simulink model "SOLTEST"  (R2026a)
settings: Solver=ode23t  StopTime=T_sweep*1.01  MaxStep=1e-3
InitFcn:
  | init_params
values from neighbouring files (symbols this model uses):
  G_cell = 1000 * ones(Ns,1)    [init_params.m]
  T_sweep = 1    [init_params.m]
  V_oc = 22.8    [init_params.m]
libraries: nesl_utility x45, pv_lib x37, fl_lib x8, ee_lib x3, simulink x2
settings Model: Creator=cdt  LastModifiedBy=cdt

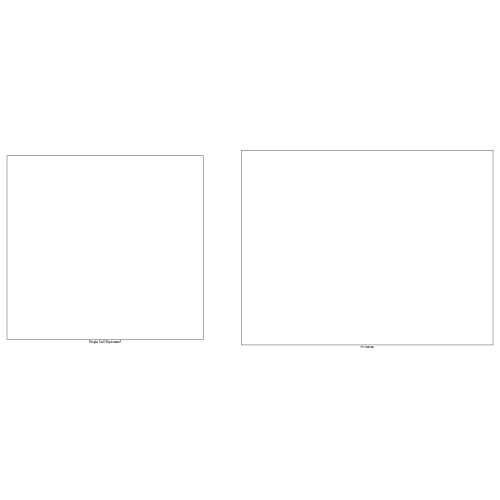
[thumbnail: Simulink's stored preview of the top-level diagram]
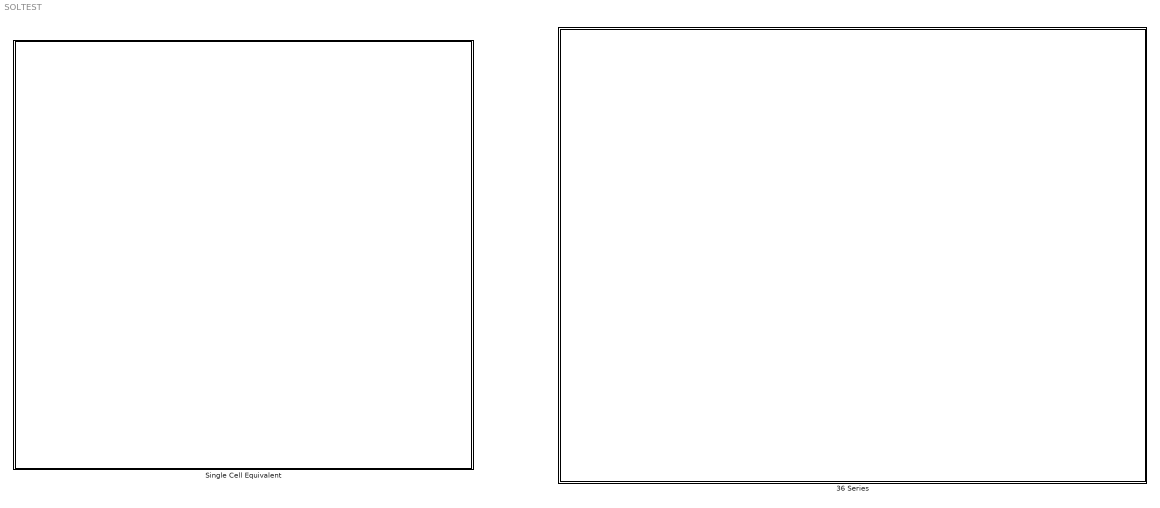
== system SOLTEST ==
  36 Series : Subsystem
  Single Cell Equivalent : Subsystem

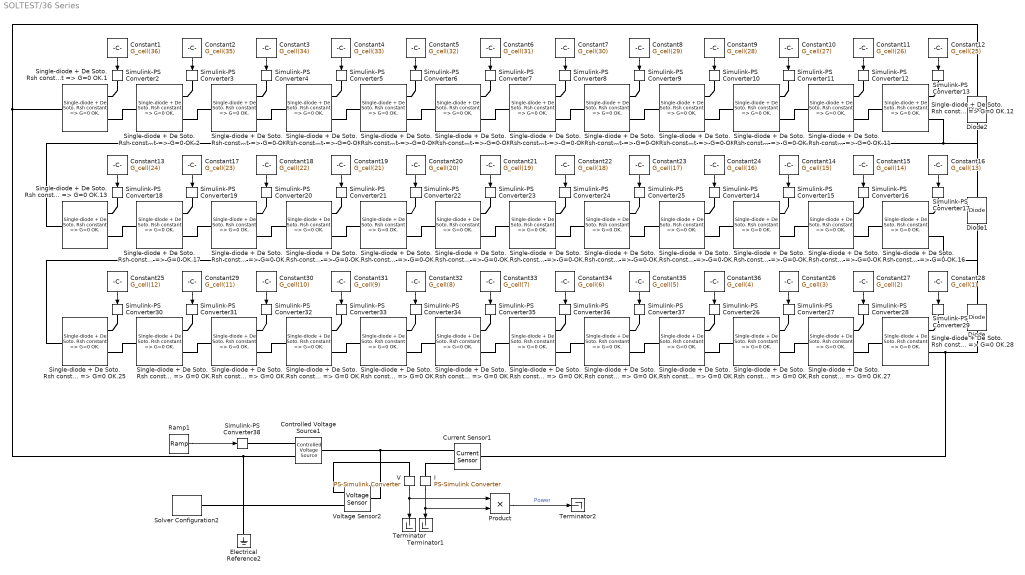
== system SOLTEST/36 Series ==
  Constant1 : Constant  Value=G_cell(36)
  Constant10 : Constant  Value=G_cell(27)
  Constant11 : Constant  Value=G_cell(26)
  Constant12 : Constant  Value=G_cell(25)
  Constant13 : Constant  Value=G_cell(24)
  Constant14 : Constant  Value=G_cell(15)
  Constant15 : Constant  Value=G_cell(14)
  Constant16 : Constant  Value=G_cell(13)
  Constant17 : Constant  Value=G_cell(23)
  Constant18 : Constant  Value=G_cell(22)
  Constant19 : Constant  Value=G_cell(21)
  Constant2 : Constant  Value=G_cell(35)
  Constant20 : Constant  Value=G_cell(20)
  Constant21 : Constant  Value=G_cell(19)
  Constant22 : Constant  Value=G_cell(18)
  Constant23 : Constant  Value=G_cell(17)
  Constant24 : Constant  Value=G_cell(16)
  Constant25 : Constant  Value=G_cell(12)
  Constant26 : Constant  Value=G_cell(3)
  Constant27 : Constant  Value=G_cell(2)
  Constant28 : Constant  Value=G_cell(1)
  Constant29 : Constant  Value=G_cell(11)
  Constant3 : Constant  Value=G_cell(34)
  Constant30 : Constant  Value=G_cell(10)
  Constant31 : Constant  Value=G_cell(9)
  Constant32 : Constant  Value=G_cell(8)
  Constant33 : Constant  Value=G_cell(7)
  Constant34 : Constant  Value=G_cell(6)
  Constant35 : Constant  Value=G_cell(5)
  Constant36 : Constant  Value=G_cell(4)
  Constant4 : Constant  Value=G_cell(33)
  Constant5 : Constant  Value=G_cell(32)
  Constant6 : Constant  Value=G_cell(31)
  Constant7 : Constant  Value=G_cell(30)
  Constant8 : Constant  Value=G_cell(29)
  Constant9 : Constant  Value=G_cell(28)
  Controlled Voltage Source1 : fl_lib/Electrical/Electrical Sources/Controlled Voltage Source
  Current Sensor1 : fl_lib/Electrical/Electrical Sensors/Current Sensor
  Diode : ee_lib/Semiconductors & Converters/Diode  ModelType=ee.enum.diode.modelType.pwl  TableType=ee.enum.diode.tableType.IfMat  IfMat=[.07, .12, .19, 1.75, 4.24, 7.32, 11.2; .16, .3, .72, 2.14, 5.02, 8.35, 13.12] A  VfMat=[.9, 1.15, 1.25, 1.5, 1.75, 2.17, 2.6, 2.85; .58, .68, .75, 1.1, 1.38, 1.77, 2.27, 2.7] V  TjVec=[25, 125] degC  VfVec=[.5, .7, .9, 1.3, 1.7, 2.1, 2.5] V  IfVec=[.1, .2, .5, 1, 2, 4, 7, 10] A  IrMat=[1e-06, 2e-06, 5e-06, 1e-05, 2.5e-05, 5e-05, .0001; 2e-06, 5e-06, 1e-05, 4e-05, 8e-05, .0002, .0005] A  VrMat=[10, 100, 200, 250, 300, 325, 350; 10, 70, 160, 220, 270, 300, 320] V  VrVec=[10, 20, 40, 50, 70, 80, 100] V  IrVec=[1e-06, 2e-06, 5e-06, 1e-05, 2e-05, 5e-05, .0001] A  Vf=0.2 V  Ron=0.3 Ohm  Goff=1e-8 S  prmExp=ee.enum.diode.expParam.useTwo  I12=[.0137, .545] A  V12=[.6, .7] V  RS=0 Ohm  Tmeas=298.15 K  IS=1e-12 A  ec=1  I1=0.0137 A  V1=0.6 V  N_series=1  N_parallel=1  ZenerEnable=false  Rz=0.3 Ohm  BV=30 V  C_param=ee.enum.diode.capParam.fixed  CJ=0 pF  CJ0=5 pF  Vvec=[.1, 10, 100] V  Cvec=[3.5, 1, .4] pF  VJ=1 V  Mgrad=0.5  FC=0.5  Q_param=ee.enum.diode.recoveryParam.off  iRM=-7.15 A  iF=4 A  didt=-750 A/us  trr_factor=3  trr=115 ns  Qrr=150 nA*s  Vr=-600 V  Ls=150 nH  Erec=0.03 J  TT=50 ns  tau=100 ns  T_param=ee.enum.diode.temperatureParam.off  Tdevice=298.15 K  I1_T2=0.245 A  V1_T2=0.5 V  IS_T2=1.25e-7 A  Tmeas2=125 degC  XTI_param=ee.enum.diode.xtiParam.pn  XTI=3  EG_param=ee.enum.diode.egapParam.material_si  EG=1.11 eV  dBVdT=0 V/K  enable_fault_input=simscape.enum.onoff.off  i_specify=off  i_priority=None  i=0 A  i_nominal_specify=off  i_nominal_value=1  i_nominal_unit=A  v_specify=off  v_priority=None  v=0 V  v_nominal_specify=off  v_nominal_value=1  v_nominal_unit=V  v_capacitor_specify=off  v_capacitor_priority=None  v_capacitor=0 V  v_capacitor_nominal_specify=off  v_capacitor_nominal_value=1  v_capacitor_nominal_unit=V  Qj_specify=off  Qj_priority=High  Qj=0 C  Qj_nominal_specify=off  Qj_nominal_value=1  Qj_nominal_unit=C  i_diode_specify=off  i_diode_priority=None  i_diode=0 A  i_diode_nominal_specify=off  i_diode_nominal_value=1  i_diode_nominal_unit=A  v_diode_specify=off  v_diode_priority=None  v_diode=0 V  v_diode_nominal_specify=off  v_diode_nominal_value=1  v_diode_nominal_unit=V  i_capacitor_specify=off  i_capacitor_priority=None  i_capacitor=0 A  i_capacitor_nominal_specify=off  i_capacitor_nominal_value=1  i_capacitor_nominal_unit=A  fidelity_level=ee.enum.diode.fidelity.includeChargeDyn  rec_loss_model=ee.enum.diode.reverseRecoveryModelTabulateUpTo3D.fixed  ErecVal=0 J  scaleWithIandV=true  ErecMat=zeros(2, 3) J  ErecMat3D=zeros(2, 3, 2) J  TjrecVec=[298.15, 398.15] K  IfrecVec=[.1, 1, 10] A  IrecVal=10 A  VrecVal=10 V  VrecVec=[0, 100] V  tFilter=1 / 1000 / 100 s  thermal_network_parameterization=ee.enum.thermalNetworkTopology.junctionCase  Rth=[0, 10] K/W  Rth_Cauer=[1, 3, 10] K/W  Rth_Foster=[.08, .14, .22, .16] K/W  thermal_mass_parameterization=ee.enum.thermalNetwork.timeconstant  thermal_mass=[0, 1] J/K  thermal_mass_Cauer=[.1, .3, 1] J/K  thermal_mass_Foster=[.001, .005, .05, .5] J/K  thermal_time_constant=[0, 10] s  thermal_time_constant_Cauer=[1, 3, 10] s  thermal_time_constant_Foster=[7e-05, .0007, .01, .08] s  thermal_mass_initial_temperatures=[25, 25] degC  thermal_mass_initial_temperatures_Cauer=[25, 25, 25] degC  junction_thermal_mass=0.01 J/K  Tvec_initial_Foster=[25, 25, 25, 25] degC  no_thermal_network=0  junction_temperature_specify=off  junction_temperature_priority=None  junction_temperature=25 degC  junction_temperature_nominal_specify=off  junction_temperature_nominal_value=1  junction_temperature_nominal_unit=degC
  Diode1 : ee_lib/Semiconductors & Converters/Diode  ModelType=ee.enum.diode.modelType.pwl  TableType=ee.enum.diode.tableType.IfMat  IfMat=[.07, .12, .19, 1.75, 4.24, 7.32, 11.2; .16, .3, .72, 2.14, 5.02, 8.35, 13.12] A  VfMat=[.9, 1.15, 1.25, 1.5, 1.75, 2.17, 2.6, 2.85; .58, .68, .75, 1.1, 1.38, 1.77, 2.27, 2.7] V  TjVec=[25, 125] degC  VfVec=[.5, .7, .9, 1.3, 1.7, 2.1, 2.5] V  IfVec=[.1, .2, .5, 1, 2, 4, 7, 10] A  IrMat=[1e-06, 2e-06, 5e-06, 1e-05, 2.5e-05, 5e-05, .0001; 2e-06, 5e-06, 1e-05, 4e-05, 8e-05, .0002, .0005] A  VrMat=[10, 100, 200, 250, 300, 325, 350; 10, 70, 160, 220, 270, 300, 320] V  VrVec=[10, 20, 40, 50, 70, 80, 100] V  IrVec=[1e-06, 2e-06, 5e-06, 1e-05, 2e-05, 5e-05, .0001] A  Vf=0.2 V  Ron=0.3 Ohm  Goff=1e-8 S  prmExp=ee.enum.diode.expParam.useTwo  I12=[.0137, .545] A  V12=[.6, .7] V  RS=0 Ohm  Tmeas=298.15 K  IS=1e-12 A  ec=1  I1=0.0137 A  V1=0.6 V  N_series=1  N_parallel=1  ZenerEnable=false  Rz=0.3 Ohm  BV=30 V  C_param=ee.enum.diode.capParam.fixed  CJ=0 pF  CJ0=5 pF  Vvec=[.1, 10, 100] V  Cvec=[3.5, 1, .4] pF  VJ=1 V  Mgrad=0.5  FC=0.5  Q_param=ee.enum.diode.recoveryParam.off  iRM=-7.15 A  iF=4 A  didt=-750 A/us  trr_factor=3  trr=115 ns  Qrr=150 nA*s  Vr=-600 V  Ls=150 nH  Erec=0.03 J  TT=50 ns  tau=100 ns  T_param=ee.enum.diode.temperatureParam.off  Tdevice=298.15 K  I1_T2=0.245 A  V1_T2=0.5 V  IS_T2=1.25e-7 A  Tmeas2=125 degC  XTI_param=ee.enum.diode.xtiParam.pn  XTI=3  EG_param=ee.enum.diode.egapParam.material_si  EG=1.11 eV  dBVdT=0 V/K  enable_fault_input=simscape.enum.onoff.off  i_specify=off  i_priority=None  i=0 A  i_nominal_specify=off  i_nominal_value=1  i_nominal_unit=A  v_specify=off  v_priority=None  v=0 V  v_nominal_specify=off  v_nominal_value=1  v_nominal_unit=V  v_capacitor_specify=off  v_capacitor_priority=None  v_capacitor=0 V  v_capacitor_nominal_specify=off  v_capacitor_nominal_value=1  v_capacitor_nominal_unit=V  Qj_specify=off  Qj_priority=High  Qj=0 C  Qj_nominal_specify=off  Qj_nominal_value=1  Qj_nominal_unit=C  i_diode_specify=off  i_diode_priority=None  i_diode=0 A  i_diode_nominal_specify=off  i_diode_nominal_value=1  i_diode_nominal_unit=A  v_diode_specify=off  v_diode_priority=None  v_diode=0 V  v_diode_nominal_specify=off  v_diode_nominal_value=1  v_diode_nominal_unit=V  i_capacitor_specify=off  i_capacitor_priority=None  i_capacitor=0 A  i_capacitor_nominal_specify=off  i_capacitor_nominal_value=1  i_capacitor_nominal_unit=A  fidelity_level=ee.enum.diode.fidelity.includeChargeDyn  rec_loss_model=ee.enum.diode.reverseRecoveryModelTabulateUpTo3D.fixed  ErecVal=0 J  scaleWithIandV=true  ErecMat=zeros(2, 3) J  ErecMat3D=zeros(2, 3, 2) J  TjrecVec=[298.15, 398.15] K  IfrecVec=[.1, 1, 10] A  IrecVal=10 A  VrecVal=10 V  VrecVec=[0, 100] V  tFilter=1 / 1000 / 100 s  thermal_network_parameterization=ee.enum.thermalNetworkTopology.junctionCase  Rth=[0, 10] K/W  Rth_Cauer=[1, 3, 10] K/W  Rth_Foster=[.08, .14, .22, .16] K/W  thermal_mass_parameterization=ee.enum.thermalNetwork.timeconstant  thermal_mass=[0, 1] J/K  thermal_mass_Cauer=[.1, .3, 1] J/K  thermal_mass_Foster=[.001, .005, .05, .5] J/K  thermal_time_constant=[0, 10] s  thermal_time_constant_Cauer=[1, 3, 10] s  thermal_time_constant_Foster=[7e-05, .0007, .01, .08] s  thermal_mass_initial_temperatures=[25, 25] degC  thermal_mass_initial_temperatures_Cauer=[25, 25, 25] degC  junction_thermal_mass=0.01 J/K  Tvec_initial_Foster=[25, 25, 25, 25] degC  no_thermal_network=0  junction_temperature_specify=off  junction_temperature_priority=None  junction_temperature=25 degC  junction_temperature_nominal_specify=off  junction_temperature_nominal_value=1  junction_temperature_nominal_unit=degC
  Diode2 : ee_lib/Semiconductors & Converters/Diode  ModelType=ee.enum.diode.modelType.pwl  TableType=ee.enum.diode.tableType.IfMat  IfMat=[.07, .12, .19, 1.75, 4.24, 7.32, 11.2; .16, .3, .72, 2.14, 5.02, 8.35, 13.12] A  VfMat=[.9, 1.15, 1.25, 1.5, 1.75, 2.17, 2.6, 2.85; .58, .68, .75, 1.1, 1.38, 1.77, 2.27, 2.7] V  TjVec=[25, 125] degC  VfVec=[.5, .7, .9, 1.3, 1.7, 2.1, 2.5] V  IfVec=[.1, .2, .5, 1, 2, 4, 7, 10] A  IrMat=[1e-06, 2e-06, 5e-06, 1e-05, 2.5e-05, 5e-05, .0001; 2e-06, 5e-06, 1e-05, 4e-05, 8e-05, .0002, .0005] A  VrMat=[10, 100, 200, 250, 300, 325, 350; 10, 70, 160, 220, 270, 300, 320] V  VrVec=[10, 20, 40, 50, 70, 80, 100] V  IrVec=[1e-06, 2e-06, 5e-06, 1e-05, 2e-05, 5e-05, .0001] A  Vf=0.2 V  Ron=0.3 Ohm  Goff=1e-8 S  prmExp=ee.enum.diode.expParam.useTwo  I12=[.0137, .545] A  V12=[.6, .7] V  RS=0 Ohm  Tmeas=298.15 K  IS=1e-12 A  ec=1  I1=0.0137 A  V1=0.6 V  N_series=1  N_parallel=1  ZenerEnable=false  Rz=0.3 Ohm  BV=30 V  C_param=ee.enum.diode.capParam.fixed  CJ=0 pF  CJ0=5 pF  Vvec=[.1, 10, 100] V  Cvec=[3.5, 1, .4] pF  VJ=1 V  Mgrad=0.5  FC=0.5  Q_param=ee.enum.diode.recoveryParam.off  iRM=-7.15 A  iF=4 A  didt=-750 A/us  trr_factor=3  trr=115 ns  Qrr=150 nA*s  Vr=-600 V  Ls=150 nH  Erec=0.03 J  TT=50 ns  tau=100 ns  T_param=ee.enum.diode.temperatureParam.off  Tdevice=298.15 K  I1_T2=0.245 A  V1_T2=0.5 V  IS_T2=1.25e-7 A  Tmeas2=125 degC  XTI_param=ee.enum.diode.xtiParam.pn  XTI=3  EG_param=ee.enum.diode.egapParam.material_si  EG=1.11 eV  dBVdT=0 V/K  enable_fault_input=simscape.enum.onoff.off  i_specify=off  i_priority=None  i=0 A  i_nominal_specify=off  i_nominal_value=1  i_nominal_unit=A  v_specify=off  v_priority=None  v=0 V  v_nominal_specify=off  v_nominal_value=1  v_nominal_unit=V  v_capacitor_specify=off  v_capacitor_priority=None  v_capacitor=0 V  v_capacitor_nominal_specify=off  v_capacitor_nominal_value=1  v_capacitor_nominal_unit=V  Qj_specify=off  Qj_priority=High  Qj=0 C  Qj_nominal_specify=off  Qj_nominal_value=1  Qj_nominal_unit=C  i_diode_specify=off  i_diode_priority=None  i_diode=0 A  i_diode_nominal_specify=off  i_diode_nominal_value=1  i_diode_nominal_unit=A  v_diode_specify=off  v_diode_priority=None  v_diode=0 V  v_diode_nominal_specify=off  v_diode_nominal_value=1  v_diode_nominal_unit=V  i_capacitor_specify=off  i_capacitor_priority=None  i_capacitor=0 A  i_capacitor_nominal_specify=off  i_capacitor_nominal_value=1  i_capacitor_nominal_unit=A  fidelity_level=ee.enum.diode.fidelity.includeChargeDyn  rec_loss_model=ee.enum.diode.reverseRecoveryModelTabulateUpTo3D.fixed  ErecVal=0 J  scaleWithIandV=true  ErecMat=zeros(2, 3) J  ErecMat3D=zeros(2, 3, 2) J  TjrecVec=[298.15, 398.15] K  IfrecVec=[.1, 1, 10] A  IrecVal=10 A  VrecVal=10 V  VrecVec=[0, 100] V  tFilter=1 / 1000 / 100 s  thermal_network_parameterization=ee.enum.thermalNetworkTopology.junctionCase  Rth=[0, 10] K/W  Rth_Cauer=[1, 3, 10] K/W  Rth_Foster=[.08, .14, .22, .16] K/W  thermal_mass_parameterization=ee.enum.thermalNetwork.timeconstant  thermal_mass=[0, 1] J/K  thermal_mass_Cauer=[.1, .3, 1] J/K  thermal_mass_Foster=[.001, .005, .05, .5] J/K  thermal_time_constant=[0, 10] s  thermal_time_constant_Cauer=[1, 3, 10] s  thermal_time_constant_Foster=[7e-05, .0007, .01, .08] s  thermal_mass_initial_temperatures=[25, 25] degC  thermal_mass_initial_temperatures_Cauer=[25, 25, 25] degC  junction_thermal_mass=0.01 J/K  Tvec_initial_Foster=[25, 25, 25, 25] degC  no_thermal_network=0  junction_temperature_specify=off  junction_temperature_priority=None  junction_temperature=25 degC  junction_temperature_nominal_specify=off  junction_temperature_nominal_value=1  junction_temperature_nominal_unit=degC
  Electrical Reference2 : fl_lib/Electrical/Electrical Elements/Electrical Reference
  I : nesl_utility/PS-Simulink Converter  PhysicalDomain=network_engine_domain  SubClassName=ps_output  LeftPortType=input  RightPortType=output  PseudoPeriodic=off  Frequencies=[]  VectorFormat=inherit  Unit=inherit  AffineConversion=off
  Product : Product
  Ramp1 : simulink/Sources/Ramp  slope=V_oc/T_sweep  start=0  InitialOutput=0
  Simulink-PS Converter{2..37} (36 alike) : nesl_utility/Simulink-PS Converter  PhysicalDomain=network_engine_domain  SubClassName=ps_input  LeftPortType=input  RightPortType=output  PseudoPeriodic=off  Frequencies=[]  NoiseDistribution=none  NoiseParameters=[]  Unit=W/m^2  AffineConversion=off  FilteringAndDerivatives=provide  SimscapeFilterOrder=1  InputFilterTimeConstant=0.001  UdotUserProvided=0
  Simulink-PS Converter38 : nesl_utility/Simulink-PS Converter  PhysicalDomain=network_engine_domain  SubClassName=ps_input  LeftPortType=input  RightPortType=output  PseudoPeriodic=off  Frequencies=[]  NoiseDistribution=none  NoiseParameters=[]  Unit=1  AffineConversion=off  FilteringAndDerivatives=provide  SimscapeFilterOrder=1  InputFilterTimeConstant=0.001  UdotUserProvided=0
  Single-diode + De Soto. Rsh constant => G=0 OK.{1..36} (36 alike) : pv_lib/Single-diode + De Soto. Rsh constant => G=0 OK.  IL_ref=IL_ref A  I0_ref=I0_ref A  a_ref=a_ref V  Rs=Rs Ohm  Rsh_ref=Rsh_ref Ohm  alpha=alpha A/K  T=298.15 K  Gref=1000 W/m^2  Tref=298.15 K  Eg_ref=1.121 eV  dEgdT=0.0002677 1/K  kB=8.617333262e-5 eV/K  i_specify=off  i_priority=None  i=0 A  i_nominal_specify=off  i_nominal_value=1  i_nominal_unit=A  v_specify=off  v_priority=None  v=0 V  v_nominal_specify=off  v_nominal_value=1  v_nominal_unit=V
  Solver Configuration2 : nesl_utility/Solver Configuration  PhysicalDomain=network_engine_domain  SubClassName=solver  LeftPortType=input  RightPortType=generic  Tones=[]  Harmonics=[]  SimulateNoise=off  Profile=off  UseLocalSampling=off  EnableSwitchedLinearOptims=on  FrequencyDomain=off  UseCCode=off  RelTol=0.001  AbsTol=0.001  MinStep=1e-09  ToWorkspace=off  RevertToSquareIcSolve=off  NumHomotopyIterations=100  PhasorMode=off  PhasorModeNumHarmonics=1  ConsistencySolver=NEWTON_XTOL_AFTER_FTOL  CanonicalOrdering=CANONICAL  OptimizeIntermediates=OPTIMIZED  IndexReductionMethod=DerivativeReplacement  DoDC=off  ResidualTolerance=1e-09  ConsistencyTolSource=GLOBAL  ConsistencyAbsTol=0.001  ConsistencyRelTol=0.001  ConsistencyTolFactor=0.001  UseLocalSolver=off  LocalSolverChoice=NE_BACKWARD_EULER_ADVANCER  ResolveIndetEquations=on  FunctionEvalNumThread=1  LocalSolverSampleTime=0.001  DoFixedCost=off  MaxNonlinIter=3  MaxModeIter=2  ComputeImpulses=off  ImpulseIterations=2  LinearAlgebra=auto  LinearAlgebraNumThread=0  EquationFormulation=NE_TIME_EF  DelaysMemoryBudget=1024  AutomaticFiltering=on  FilteringTimeConstant=0.001  PartitionStorageMethod=AS_NEEDED  PartitionMemoryBudget=1024  PartitionMethod=ROBUST  MultibodyUseLocalSolver=off  MultibodyLocalSolverChoice=ODE1  MultibodyLocalSolverSampleTime=0.001
  Terminator : Terminator
  Terminator1 : Terminator
  Terminator2 : Terminator
  V : nesl_utility/PS-Simulink Converter  PhysicalDomain=network_engine_domain  SubClassName=ps_output  LeftPortType=input  RightPortType=output  PseudoPeriodic=off  Frequencies=[]  VectorFormat=inherit  Unit=inherit  AffineConversion=off
  Voltage Sensor2 : fl_lib/Electrical/Electrical Sensors/Voltage Sensor
  wires:
  Constant25/1 -> Simulink-PS Converter30/1
  Constant14/1 -> Simulink-PS Converter15/1
  I/1 -> Product/2, Terminator1/1
  Constant33/1 -> Simulink-PS Converter35/1
  Constant9/1 -> Simulink-PS Converter10/1
  Ramp1/1 -> Simulink-PS Converter38/1
  V/1 -> Product/1, Terminator/1
  Constant19/1 -> Simulink-PS Converter21/1
  Constant29/1 -> Simulink-PS Converter31/1
  Constant11/1 -> Simulink-PS Converter12/1
  Constant3/1 -> Simulink-PS Converter4/1
  Constant35/1 -> Simulink-PS Converter37/1
  Constant31/1 -> Simulink-PS Converter33/1
  Constant36/1 -> Simulink-PS Converter26/1
  Constant22/1 -> Simulink-PS Converter24/1
  Constant5/1 -> Simulink-PS Converter6/1
  Constant24/1 -> Simulink-PS Converter14/1
  Constant4/1 -> Simulink-PS Converter5/1
  Constant1/1 -> Simulink-PS Converter2/1
  Constant28/1 -> Simulink-PS Converter29/1
  Constant15/1 -> Simulink-PS Converter16/1
  Constant26/1 -> Simulink-PS Converter27/1
  Constant2/1 -> Simulink-PS Converter3/1
  Constant6/1 -> Simulink-PS Converter7/1
  Constant16/1 -> Simulink-PS Converter17/1
  Constant18/1 -> Simulink-PS Converter20/1
  Constant7/1 -> Simulink-PS Converter8/1
  Constant12/1 -> Simulink-PS Converter13/1
  Constant20/1 -> Simulink-PS Converter22/1
  Constant32/1 -> Simulink-PS Converter34/1
  Constant17/1 -> Simulink-PS Converter19/1
  Constant23/1 -> Simulink-PS Converter25/1
  Constant27/1 -> Simulink-PS Converter28/1
  Constant8/1 -> Simulink-PS Converter9/1
  Constant30/1 -> Simulink-PS Converter32/1
  Constant34/1 -> Simulink-PS Converter36/1
  Constant21/1 -> Simulink-PS Converter23/1
  Constant13/1 -> Simulink-PS Converter18/1
  Constant10/1 -> Simulink-PS Converter11/1
  Product/1 -> Terminator2/1  "Power"
  connections:
  Single-diode + De Soto. Rsh constant => G=0 OK.24/RConn1 -- Single-diode + De Soto. Rsh constant => G=0 OK.23/LConn1
  Simulink-PS Converter8/RConn1 -- Single-diode + De Soto. Rsh constant => G=0 OK.7/LConn2
  Single-diode + De Soto. Rsh constant => G=0 OK.17/RConn1 -- Single-diode + De Soto. Rsh constant => G=0 OK.13/LConn1
  Single-diode + De Soto. Rsh constant => G=0 OK.33/RConn1 -- Single-diode + De Soto. Rsh constant => G=0 OK.32/LConn1
  Single-diode + De Soto. Rsh constant => G=0 OK.2/RConn1 -- Single-diode + De Soto. Rsh constant => G=0 OK.1/LConn1
  Single-diode + De Soto. Rsh constant => G=0 OK.18/RConn1 -- Single-diode + De Soto. Rsh constant => G=0 OK.17/LConn1
  Simulink-PS Converter27/RConn1 -- Single-diode + De Soto. Rsh constant => G=0 OK.26/LConn2
  Simulink-PS Converter35/RConn1 -- Single-diode + De Soto. Rsh constant => G=0 OK.33/LConn2
  Single-diode + De Soto. Rsh constant => G=0 OK.22/RConn1 -- Single-diode + De Soto. Rsh constant => G=0 OK.21/LConn1
  Single-diode + De Soto. Rsh constant => G=0 OK.20/RConn1 -- Single-diode + De Soto. Rsh constant => G=0 OK.19/LConn1
  Simulink-PS Converter13/RConn1 -- Single-diode + De Soto. Rsh constant => G=0 OK.12/LConn2
  Single-diode + De Soto. Rsh constant => G=0 OK.11/RConn1 -- Single-diode + De Soto. Rsh constant => G=0 OK.10/LConn1
  Single-diode + De Soto. Rsh constant => G=0 OK.23/RConn1 -- Single-diode + De Soto. Rsh constant => G=0 OK.22/LConn1
  Simulink-PS Converter31/RConn1 -- Single-diode + De Soto. Rsh constant => G=0 OK.29/LConn2
  Simulink-PS Converter28/RConn1 -- Single-diode + De Soto. Rsh constant => G=0 OK.27/LConn2
  Single-diode + De Soto. Rsh constant => G=0 OK.3/RConn1 -- Single-diode + De Soto. Rsh constant => G=0 OK.2/LConn1
  Simulink-PS Converter2/RConn1 -- Single-diode + De Soto. Rsh constant => G=0 OK.1/LConn2
  Single-diode + De Soto. Rsh constant => G=0 OK.16/RConn1 -- Single-diode + De Soto. Rsh constant => G=0 OK.15/LConn1
  Simulink-PS Converter21/RConn1 -- Single-diode + De Soto. Rsh constant => G=0 OK.19/LConn2
  Simulink-PS Converter33/RConn1 -- Single-diode + De Soto. Rsh constant => G=0 OK.31/LConn2
  Single-diode + De Soto. Rsh constant => G=0 OK.4/RConn1 -- Single-diode + De Soto. Rsh constant => G=0 OK.3/LConn1
  Single-diode + De Soto. Rsh constant => G=0 OK.32/RConn1 -- Single-diode + De Soto. Rsh constant => G=0 OK.31/LConn1
  Single-diode + De Soto. Rsh constant => G=0 OK.29/RConn1 -- Single-diode + De Soto. Rsh constant => G=0 OK.25/LConn1
  Single-diode + De Soto. Rsh constant => G=0 OK.34/RConn1 -- Single-diode + De Soto. Rsh constant => G=0 OK.33/LConn1
  Simulink-PS Converter25/RConn1 -- Single-diode + De Soto. Rsh constant => G=0 OK.23/LConn2
  Simulink-PS Converter6/RConn1 -- Single-diode + De Soto. Rsh constant => G=0 OK.5/LConn2
  Simulink-PS Converter36/RConn1 -- Single-diode + De Soto. Rsh constant => G=0 OK.34/LConn2
  Simulink-PS Converter4/RConn1 -- Single-diode + De Soto. Rsh constant => G=0 OK.3/LConn2
  Simulink-PS Converter15/RConn1 -- Single-diode + De Soto. Rsh constant => G=0 OK.14/LConn2
  Voltage Sensor2/RConn1 -- V/LConn1
  Single-diode + De Soto. Rsh constant => G=0 OK.12/RConn1 -- Single-diode + De Soto. Rsh constant => G=0 OK.11/LConn1
  Single-diode + De Soto. Rsh constant => G=0 OK.8/RConn1 -- Single-diode + De Soto. Rsh constant => G=0 OK.7/LConn1
  I/LConn1 -- Current Sensor1/RConn1
  Simulink-PS Converter16/RConn1 -- Single-diode + De Soto. Rsh constant => G=0 OK.15/LConn2
  Simulink-PS Converter29/RConn1 -- Single-diode + De Soto. Rsh constant => G=0 OK.28/LConn2
  Simulink-PS Converter10/RConn1 -- Single-diode + De Soto. Rsh constant => G=0 OK.9/LConn2
  Single-diode + De Soto. Rsh constant => G=0 OK.28/LConn1 -- Diode/RConn1 -- Current Sensor1/LConn1
  Single-diode + De Soto. Rsh constant => G=0 OK.35/RConn1 -- Single-diode + De Soto. Rsh constant => G=0 OK.34/LConn1
  Single-diode + De Soto. Rsh constant => G=0 OK.26/RConn1 -- Single-diode + De Soto. Rsh constant => G=0 OK.36/LConn1
  Simulink-PS Converter32/RConn1 -- Single-diode + De Soto. Rsh constant => G=0 OK.30/LConn2
  Simulink-PS Converter19/RConn1 -- Single-diode + De Soto. Rsh constant => G=0 OK.17/LConn2
  Single-diode + De Soto. Rsh constant => G=0 OK.21/RConn1 -- Single-diode + De Soto. Rsh constant => G=0 OK.20/LConn1
  Simulink-PS Converter20/RConn1 -- Single-diode + De Soto. Rsh constant => G=0 OK.18/LConn2
  Controlled Voltage Source1/RConn2 -- Electrical Reference2/LConn1 -- Voltage Sensor2/RConn2 -- Solver Configuration2/RConn1 -- Diode2/LConn1 -- Single-diode + De Soto. Rsh constant => G=0 OK.1/RConn1
  Single-diode + De Soto. Rsh constant => G=0 OK.14/RConn1 -- Single-diode + De Soto. Rsh constant => G=0 OK.24/LConn1
  Simulink-PS Converter22/RConn1 -- Single-diode + De Soto. Rsh constant => G=0 OK.20/LConn2
  Simulink-PS Converter3/RConn1 -- Single-diode + De Soto. Rsh constant => G=0 OK.2/LConn2
  Single-diode + De Soto. Rsh constant => G=0 OK.31/RConn1 -- Single-diode + De Soto. Rsh constant => G=0 OK.30/LConn1
  Simulink-PS Converter26/RConn1 -- Single-diode + De Soto. Rsh constant => G=0 OK.36/LConn2
  Single-diode + De Soto. Rsh constant => G=0 OK.5/RConn1 -- Single-diode + De Soto. Rsh constant => G=0 OK.4/LConn1
  Single-diode + De Soto. Rsh constant => G=0 OK.9/RConn1 -- Single-diode + De Soto. Rsh constant => G=0 OK.8/LConn1
  Simulink-PS Converter12/RConn1 -- Single-diode + De Soto. Rsh constant => G=0 OK.11/LConn2
  Simulink-PS Converter30/RConn1 -- Single-diode + De Soto. Rsh constant => G=0 OK.25/LConn2
  Simulink-PS Converter11/RConn1 -- Single-diode + De Soto. Rsh constant => G=0 OK.10/LConn2
  Simulink-PS Converter5/RConn1 -- Single-diode + De Soto. Rsh constant => G=0 OK.4/LConn2
  Single-diode + De Soto. Rsh constant => G=0 OK.16/LConn1 -- Diode/LConn1 -- Diode1/RConn1 -- Single-diode + De Soto. Rsh constant => G=0 OK.25/RConn1
  Simulink-PS Converter37/RConn1 -- Single-diode + De Soto. Rsh constant => G=0 OK.35/LConn2
  Single-diode + De Soto. Rsh constant => G=0 OK.10/RConn1 -- Single-diode + De Soto. Rsh constant => G=0 OK.9/LConn1
  Simulink-PS Converter23/RConn1 -- Single-diode + De Soto. Rsh constant => G=0 OK.21/LConn2
  Single-diode + De Soto. Rsh constant => G=0 OK.19/RConn1 -- Single-diode + De Soto. Rsh constant => G=0 OK.18/LConn1
  Single-diode + De Soto. Rsh constant => G=0 OK.27/RConn1 -- Single-diode + De Soto. Rsh constant => G=0 OK.26/LConn1
  Single-diode + De Soto. Rsh constant => G=0 OK.30/RConn1 -- Single-diode + De Soto. Rsh constant => G=0 OK.29/LConn1
  Controlled Voltage Source1/LConn1 -- Voltage Sensor2/LConn1 -- Current Sensor1/RConn2
  Simulink-PS Converter7/RConn1 -- Single-diode + De Soto. Rsh constant => G=0 OK.6/LConn2
  Simulink-PS Converter34/RConn1 -- Single-diode + De Soto. Rsh constant => G=0 OK.32/LConn2
  Single-diode + De Soto. Rsh constant => G=0 OK.28/RConn1 -- Single-diode + De Soto. Rsh constant => G=0 OK.27/LConn1
  Simulink-PS Converter24/RConn1 -- Single-diode + De Soto. Rsh constant => G=0 OK.22/LConn2
  Simulink-PS Converter9/RConn1 -- Single-diode + De Soto. Rsh constant => G=0 OK.8/LConn2
  Single-diode + De Soto. Rsh constant => G=0 OK.7/RConn1 -- Single-diode + De Soto. Rsh constant => G=0 OK.6/LConn1
  Simulink-PS Converter17/RConn1 -- Single-diode + De Soto. Rsh constant => G=0 OK.16/LConn2
  Single-diode + De Soto. Rsh constant => G=0 OK.36/RConn1 -- Single-diode + De Soto. Rsh constant => G=0 OK.35/LConn1
  Simulink-PS Converter14/RConn1 -- Single-diode + De Soto. Rsh constant => G=0 OK.24/LConn2
  Simulink-PS Converter38/RConn1 -- Controlled Voltage Source1/RConn1
  Single-diode + De Soto. Rsh constant => G=0 OK.6/RConn1 -- Single-diode + De Soto. Rsh constant => G=0 OK.5/LConn1
  Single-diode + De Soto. Rsh constant => G=0 OK.12/LConn1 -- Diode1/LConn1 -- Diode2/RConn1 -- Single-diode + De Soto. Rsh constant => G=0 OK.13/RConn1
  Single-diode + De Soto. Rsh constant => G=0 OK.15/RConn1 -- Single-diode + De Soto. Rsh constant => G=0 OK.14/LConn1
  Simulink-PS Converter18/RConn1 -- Single-diode + De Soto. Rsh constant => G=0 OK.13/LConn2

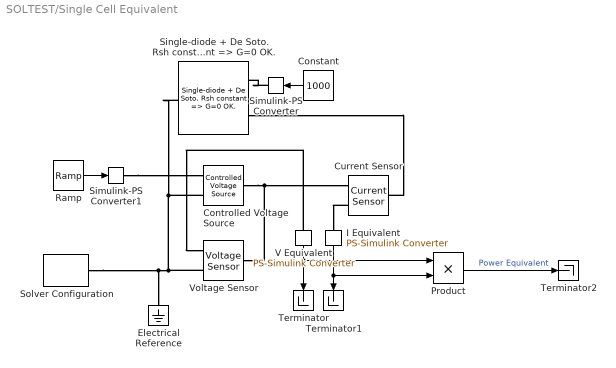
== system SOLTEST/Single Cell Equivalent ==
  Constant : Constant  Value=1000
  Controlled Voltage Source : fl_lib/Electrical/Electrical Sources/Controlled Voltage Source
  Current Sensor : fl_lib/Electrical/Electrical Sensors/Current Sensor
  Electrical Reference : fl_lib/Electrical/Electrical Elements/Electrical Reference
  I Equivalent : nesl_utility/PS-Simulink Converter  PhysicalDomain=network_engine_domain  SubClassName=ps_output  LeftPortType=input  RightPortType=output  PseudoPeriodic=off  Frequencies=[]  VectorFormat=inherit  Unit=inherit  AffineConversion=off
  Product : Product
  Ramp : simulink/Sources/Ramp  slope=V_oc/T_sweep  start=0  InitialOutput=0
  Simulink-PS Converter : nesl_utility/Simulink-PS Converter  PhysicalDomain=network_engine_domain  SubClassName=ps_input  LeftPortType=input  RightPortType=output  PseudoPeriodic=off  Frequencies=[]  NoiseDistribution=none  NoiseParameters=[]  Unit=W/m^2  AffineConversion=off  FilteringAndDerivatives=provide  SimscapeFilterOrder=1  InputFilterTimeConstant=0.001  UdotUserProvided=0
  Simulink-PS Converter1 : nesl_utility/Simulink-PS Converter  PhysicalDomain=network_engine_domain  SubClassName=ps_input  LeftPortType=input  RightPortType=output  PseudoPeriodic=off  Frequencies=[]  NoiseDistribution=none  NoiseParameters=[]  Unit=1  AffineConversion=off  FilteringAndDerivatives=provide  SimscapeFilterOrder=1  InputFilterTimeConstant=0.001  UdotUserProvided=0
  Single-diode + De Soto. Rsh constant => G=0 OK. : pv_lib/Single-diode + De Soto. Rsh constant => G=0 OK.  IL_ref=IL_m A  I0_ref=I0_m A  a_ref=a_m V  Rs=Rs_m Ohm  Rsh_ref=Rsh_m Ohm  alpha=alpha A/K  T=298.15 K  Gref=1000 W/m^2  Tref=298.15 K  Eg_ref=1.121 eV  dEgdT=0.0002677 1/K  kB=8.617333262e-5 eV/K  i_specify=off  i_priority=None  i=0 A  i_nominal_specify=off  i_nominal_value=1  i_nominal_unit=A  v_specify=off  v_priority=None  v=0 V  v_nominal_specify=off  v_nominal_value=1  v_nominal_unit=V
  Solver Configuration : nesl_utility/Solver Configuration  PhysicalDomain=network_engine_domain  SubClassName=solver  LeftPortType=input  RightPortType=generic  Tones=[]  Harmonics=[]  SimulateNoise=off  Profile=off  UseLocalSampling=off  EnableSwitchedLinearOptims=on  FrequencyDomain=off  UseCCode=off  RelTol=0.001  AbsTol=0.001  MinStep=1e-09  ToWorkspace=off  RevertToSquareIcSolve=off  NumHomotopyIterations=100  PhasorMode=off  PhasorModeNumHarmonics=1  ConsistencySolver=NEWTON_XTOL_AFTER_FTOL  CanonicalOrdering=CANONICAL  OptimizeIntermediates=OPTIMIZED  IndexReductionMethod=DerivativeReplacement  DoDC=off  ResidualTolerance=1e-09  ConsistencyTolSource=GLOBAL  ConsistencyAbsTol=0.001  ConsistencyRelTol=0.001  ConsistencyTolFactor=0.001  UseLocalSolver=off  LocalSolverChoice=NE_BACKWARD_EULER_ADVANCER  ResolveIndetEquations=on  FunctionEvalNumThread=1  LocalSolverSampleTime=0.001  DoFixedCost=off  MaxNonlinIter=3  MaxModeIter=2  ComputeImpulses=off  ImpulseIterations=2  LinearAlgebra=auto  LinearAlgebraNumThread=0  EquationFormulation=NE_TIME_EF  DelaysMemoryBudget=1024  AutomaticFiltering=on  FilteringTimeConstant=0.001  PartitionStorageMethod=AS_NEEDED  PartitionMemoryBudget=1024  PartitionMethod=ROBUST  MultibodyUseLocalSolver=off  MultibodyLocalSolverChoice=ODE1  MultibodyLocalSolverSampleTime=0.001
  Terminator : Terminator
  Terminator1 : Terminator
  Terminator2 : Terminator
  V Equivalent : nesl_utility/PS-Simulink Converter  PhysicalDomain=network_engine_domain  SubClassName=ps_output  LeftPortType=input  RightPortType=output  PseudoPeriodic=off  Frequencies=[]  VectorFormat=inherit  Unit=inherit  AffineConversion=off
  Voltage Sensor : fl_lib/Electrical/Electrical Sensors/Voltage Sensor
  wires:
  Ramp/1 -> Simulink-PS Converter1/1
  V Equivalent/1 -> Terminator/1, Product/1
  Constant/1 -> Simulink-PS Converter/1
  I Equivalent/1 -> Product/2, Terminator1/1
  Product/1 -> Terminator2/1  "Power Equivalent"
  connections:
  Current Sensor/RConn1 -- I Equivalent/LConn1
  Simulink-PS Converter/RConn1 -- Single-diode + De Soto. Rsh constant => G=0 OK./LConn2
  V Equivalent/LConn1 -- Voltage Sensor/RConn1
  Simulink-PS Converter1/RConn1 -- Controlled Voltage Source/RConn1
  Controlled Voltage Source/LConn1 -- Voltage Sensor/LConn1 -- Current Sensor/RConn2
  Single-diode + De Soto. Rsh constant => G=0 OK./LConn1 -- Current Sensor/LConn1
  Solver Configuration/RConn1 -- Voltage Sensor/RConn2 -- Single-diode + De Soto. Rsh constant => G=0 OK./RConn1 -- Controlled Voltage Source/RConn2 -- Electrical Reference/LConn1
